simulink model "mPortSampleTime"  (Simulink 7.1)
settings: Solver=FixedStepDiscrete  StartTime=0.0  StopTime=inf  RelTol=1e-3
undefined symbols (not defined in the file or in its folder): paramIn, paramOut
settings Model: Creator=jcobleig  LastModifiedBy=jcobleig
settings OptimizationCC: InlineParams=on
settings DebuggingCC: StrictBusMsg=ErrorLevel1

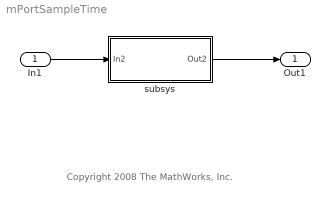
== system mPortSampleTime ==
  note: Copyright 2008 The MathWorks, Inc.
  In1 : Inport  OutDataType=sfix(16)  OutScaling=2^0
      settings: AttributesFormatString=st = %<SampleTime>
  subsys : Subsystem  TreatAsAtomicUnit=on
  Out1 : Outport  OutDataType=sfix(16)  OutScaling=2^0
  wires:
  In1/1 -> subsys/1(In2)
  subsys/1(Out2) -> Out1/1

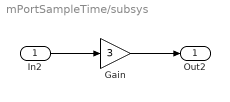
== system mPortSampleTime/subsys ==
  In2 : Inport  SampleTime=paramIn  OutDataType=sfix(16)  OutScaling=2^0
      settings: AttributesFormatString=st = %<SampleTime>
  Gain : Gain  Gain=3  ParameterDataType=sfix(16)  ParameterScaling=2^0  OutDataType=sfix(16)  OutScaling=2^0
  Out2 : Outport  SampleTime=paramOut  OutDataType=sfix(16)  OutScaling=2^0
      settings: AttributesFormatString=st = %<SampleTime>
  wires:
  In2/1 -> Gain/1
  Gain/1 -> Out2/1
